simulink model "Planar_robot_2DoF_sim"  (R2023a)
settings: Solver=ode3  StartTime=0.0  StopTime=100  FixedStep=0.001  RelTol=1e-3
undefined symbols (not defined in the file): amplitude, arm_length, freq, radius, rho
settings Model: Creator=wu_xw  LastModifiedBy=divij
settings SolverCC: AlgebraicLoopSolver=TrustRegion
settings DataIOCC: SaveFormat=Structure  SaveOutput=off  SignalLogging=off  DSMLogging=off  SaveTime=off  ReturnWorkspaceOutputs=off
settings OptimizationCC: DefaultParameterBehavior=Inlined  UseDivisionForNetSlopeComputation=on  GainParamInheritBuiltInType=on  UseFloatMulNetSlope=on  InlineInvariantSignals=on  ZeroExternalMemoryAtStartup=off  ZeroInternalMemoryAtStartup=off  EfficientFloat2IntCast=on  LifeSpan=1  OptimizeDataStoreBuffers=off  BusAssignmentInplaceUpdate=off
settings DebuggingCC: UnconnectedInputMsg=warning  UnconnectedOutputMsg=warning  UnconnectedLineMsg=warning  SFUnexpectedBacktrackingDiag=warning  SFNoUnconditionalDefaultTransitionDiag=warning  ArithmeticOperatorsInVariantConditions=warning
settings HardwareCC: ProdLongLongMode=on
settings ModelReferenceCC: EnableRefExpFcnMdlSchedulingChecks=on
settings SFSimCC: SimUseLocalCustomCode=off  MATLABDynamicMemAlloc=off  CustomCodeUndefinedFunction=UseInterfaceOnly
settings RTWCC: GenCodeOnly=on  PackageGeneratedCodeAndArtifacts=on  GenerateReport=on  RTWUseLocalCustomCode=off  Toolchain=Catkin  BuildConfiguration=Debug  LaunchReport=on  TargetLang=C++
settings CodeAppCC: ForceParamTrailComments=on  EnableCustomComments=on
settings GRTTargetCC: TargetLangStandard=C++11 (ISO)  CombineSignalStateStructs=on  MatFileLogging=off  CodeInterfacePackaging=C++ class  SupportVariableSizeSignals=on  MultiInstanceErrorCode=Warning

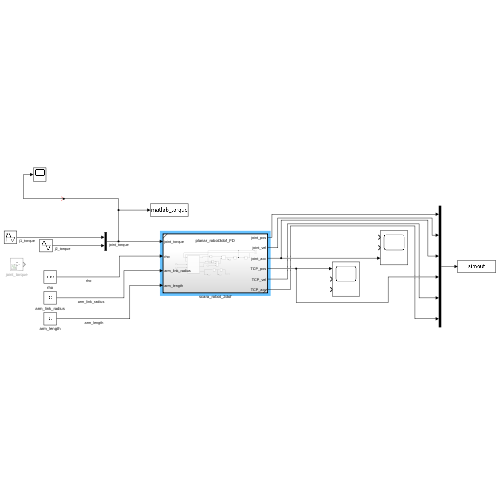
[thumbnail: Simulink's stored preview of the top-level diagram]
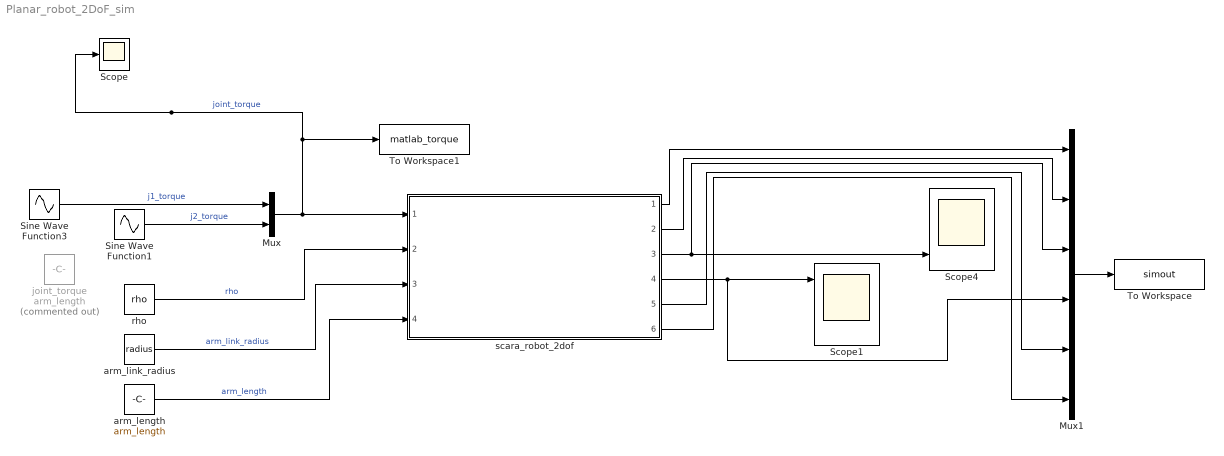
== system Planar_robot_2DoF_sim ==
  Mux : Mux  Inputs=2
  Mux1 : Mux  Inputs=6
  Scope : Scope
  Scope1 : Scope  NumInputPorts=3
  Scope4 : Scope  NumInputPorts=3
  Sine Wave Function1 : Sin  Amplitude=amplitude(2)  Frequency=freq(2)  SampleTime=0
  Sine Wave Function3 : Sin  Amplitude=amplitude(1)  Frequency=freq(1)  SampleTime=0
  To Workspace : ToWorkspace  VariableName=simout  SaveFormat=Structure  SampleTime=-1
  To Workspace1 : ToWorkspace  VariableName=matlab_torque  SampleTime=-1
      settings: Save2DSignal=2-D array (concatenate along first dimension)
  arm_length : Constant  Value=arm_length  SampleTime=-1
  arm_link_radius : Constant  Value=radius  SampleTime=-1
  joint_torque : Constant  Commented=on  Value=arm_length  SampleTime=-1
  rho : Constant  Value=rho  SampleTime=-1
  scara_robot_2dof : Subsystem  TreatAsAtomicUnit=on  ReferencedSubsystem=planar_robot3dof_FD
  wires:
  Sine Wave Function1/1 -> Mux/2  "j2_torque"
  arm_length/1 -> scara_robot_2dof/4  "arm_length"
  rho/1 -> scara_robot_2dof/2  "rho"
  arm_link_radius/1 -> scara_robot_2dof/3  "arm_link_radius"
  Mux/1 -> Scope/1, To Workspace1/1, scara_robot_2dof/1  "joint_torque"
  scara_robot_2dof/1 -> Mux1/1
  scara_robot_2dof/2 -> Mux1/2
  scara_robot_2dof/3 -> Scope4/3, Mux1/3
  scara_robot_2dof/4 -> Scope1/1, Mux1/4
  scara_robot_2dof/5 -> Mux1/5
  scara_robot_2dof/6 -> Mux1/6
  Mux1/1 -> To Workspace/1
  Sine Wave Function3/1 -> Mux/1  "j1_torque"
